simulink model "Elec_stim_model"  (R2017a)
settings: Solver=FixedStepDiscrete  StartTime=0.0  StopTime=inf  FixedStep=1/500  RelTol=1e-3  EnableMultiTasking=on
StopFcn:
  | AutoStartBatchData=load('session1.mat');AutoStartBatchData=AutoStartBatchData.y;run('AEP_P300_Evaluation')
model workspace (MAT data in the model file):
  cfg_native : struct (value not decoded)
  en_add_channels = 1
  host_ip = 2130706433
  host_port = 50223
  local_ip = 2130706433
  local_port = 50224
  num_en_channels = 32
  num_samples = 8
  sample_rate = 500
  serial_number = 'NR-2018.09.02'
undefined symbols (not defined in the file): NR
libraries: gtecHighspeedLib x2, gNautilusLib x1
settings Model: Creator=Holzner  LastModifiedBy=user
settings DataIOCC: LimitDataPoints=on  SaveFormat=Array
settings OptimizationCC: LifeSpan=inf
settings DebuggingCC: UnderspecifiedInitializationDetection=Classic  MergeDetectMultiDrivingBlocksExec=none  SolverPrmCheckMsg=warning  FrameProcessingCompatibilityMsg=none  StateNameClashWarn=warning  SFUnexpectedBacktrackingDiag=warning  SFNoUnconditionalDefaultTransitionDiag=warning  SFExecutionAtInitializationDiag=none
settings HardwareCC: ProdBitPerPointer=32  ProdBitPerSizeT=32  ProdBitPerPtrDiffT=32  ProdLargestAtomicFloat=None  ProdIntDivRoundTo=Undefined  ProdEndianess=Unspecified  ProdWordSize=32  ProdHWDeviceType=32-bit Generic
settings ModelReferenceCC: PropagateSignalLabelsOutOfModel=off
settings GRTTargetCC: TargetLangStandard=C89/C90 (ANSI)  GeneratePreprocessorConditionals=Disable all
settings ConfigComp: CovMetricSettings=dw  CovHtmlReporting=on  CovSaveCumulativeToWorkspaceVar=on  CovSaveSingleToWorkspaceVar=on  CovExternalEMLEnable=off  CovSFcnEnable=off

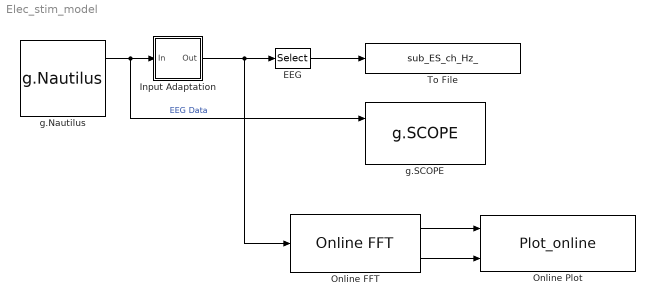
== system Elec_stim_model ==
  EEG : Selector  InputPortWidth=32  IndexOptions=Index vector (dialog)  Indices=[1:32]  OutputSizes=1
  Input Adaptation : Subsystem
  Online FFT : gtecHighspeedLib/Online FFT  fftLength=1000  fftType_select=FFT  fftType=0  windowType_select=BOXCAR  windowType=2  overlap=0  average=1
      settings: SourceProductName=g.tec Highspeed Library
  Online Plot : M-S-Function  AncestorBlock=gtecHighspeedLib185/Online Plot  FunctionName=Plot_online  Parameters=channels,xaxis,yaxis,pretrigger,evenodd,twocolmode,x_label  mask(Online Plot){channels=[1  2  3  4  5  6  7  8  9], xaxis=[], x_label=Normalized Frequency, yaxis=[0  20], pretrigger=0, evenodd=off, twocolmode=off}
      mask prompts: channels "Channels (int vector)"; xaxis "x - scale ([xmin,xmax] or [] for 'auto')"; x_label "x - label"; yaxis "y - scale ([ymin,ymax] or [] for 'auto')"; pretrigger "Pretrigger [s]"; evenodd "Show separate averages for add and even trials"; twocolmode "Two columns mode"
      mask help: This block plots the results of the online blocks.
      settings: OpenFcn=OpenAveragePlot(gcbh);
      mask Help: web(['file:///' which('gtecHS.htm')],'-helpbrowser');
      mask TypeOptions x_label: Time in sec | Normalized Frequency
      mask Display:
      | disp('Online \n Plot');
      | port_label('input',1,'Input Data');
  To File : ToFile  Filename=sub_ES_ch_Hz_  MatrixName=y
  g.Nautilus : gNautilusLib/g.Nautilus  Tag=g.Nautilus  Description=Operates a g.Nautilus device and provides acquired data on its outputs.  sample_rate=500  local_ip=2130706433  local_port=50224  host_ip=2130706433  host_port=50223  serial_number=NR-2018.09.02  num_samples=8  num_en_channels=32  add_channels=1
      settings: SourceProductName=g.Nautilus
  g.SCOPE : gtecHighspeedLib/g.SCOPE
      settings: SourceProductName=g.tec Highspeed Library
  wires:
  g.Nautilus/1 -> g.SCOPE/1, Input Adaptation/1(In)  "EEG Data"
  Input Adaptation/1(Out) -> Online FFT/1, EEG/1
  EEG/1 -> To File/1
  Online FFT/1 -> Online Plot/1
  Online FFT/2 -> Online Plot/2

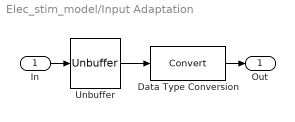
== system Elec_stim_model/Input Adaptation ==
  In : Inport  OutDataTypeStr=single
  Data Type Conversion : DataTypeConversion
  Unbuffer : Unbuffer
  Out : Outport
  wires:
  In/1 -> Unbuffer/1
  Unbuffer/1 -> Data Type Conversion/1
  Data Type Conversion/1 -> Out/1
